simulink model "Tarea2Simulacion"  (R2025a)
settings: Solver=ode8  StartTime=0.0  StopTime=1  RelTol=1e-3
settings Model: Creator=440G5  LastModifiedBy=440G5

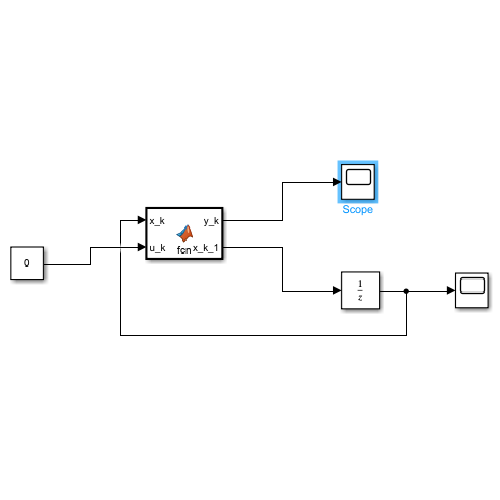
[thumbnail: Simulink's stored preview of the top-level diagram]
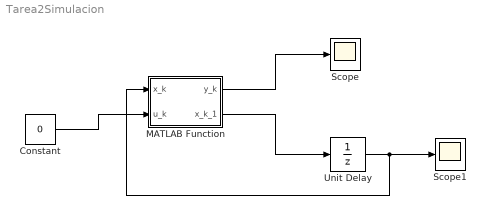
== system Tarea2Simulacion ==
  Constant : Constant  Value=0
  MATLAB Function : MATLAB Function  TreatAsAtomicUnit=on
  Scope : Scope
      settings: ActiveDisplayYMinimum=-0.31070071263664883  ActiveDisplayYMaximum=0.47897122341823906
  Scope1 : Scope
      settings: ActiveDisplayYMinimum=-0.2625  ActiveDisplayYMaximum=0.36249999999999993
  Unit Delay : UnitDelay  InitialCondition=[0.2; 0.1; 0.3]  SampleTime=-1  HasFrameUpgradeWarning=on
  wires:
  Constant/1 -> MATLAB Function/2(u_k)
  MATLAB Function/2(x_k_1) -> Unit Delay/1
  MATLAB Function/1(y_k) -> Scope/1
  Unit Delay/1 -> Scope1/1, MATLAB Function/1(x_k)

== matlab function Tarea2Simulacion/MATLAB Function ==
  data: x_k input; y_k output; u_k input; x_k_1 output
function [y_k, x_k_1] = fcn(x_k, u_k)

A = (-2/3)*[1 1 0; 0 1 0; -1 1 1];
B = [0; 1; 0];
C = [1 0 0];
x_k_1 = A*x_k + B*u_k;
y_k = C*x_k;
